simulink model "RO"  (R2023a)
settings: Solver=VariableStepAuto  StartTime=0.0  StopTime=10.0  RelTol=1e-3
undefined symbols (not defined in the file): SR
settings Model: Creator=mekala.suresh  LastModifiedBy=andres.lucht
settings OptimizationCC: ReuseModelBlockBuffer=off

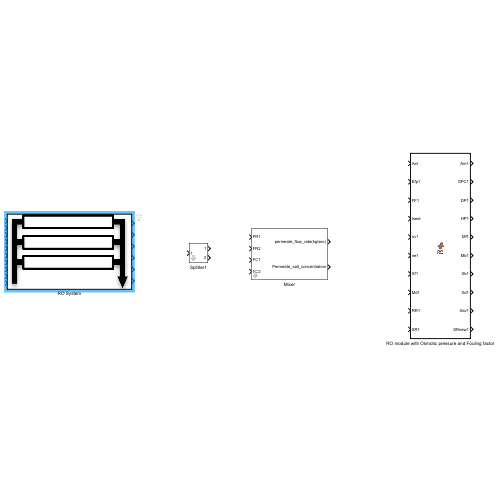
[thumbnail: Simulink's stored preview of the top-level diagram]
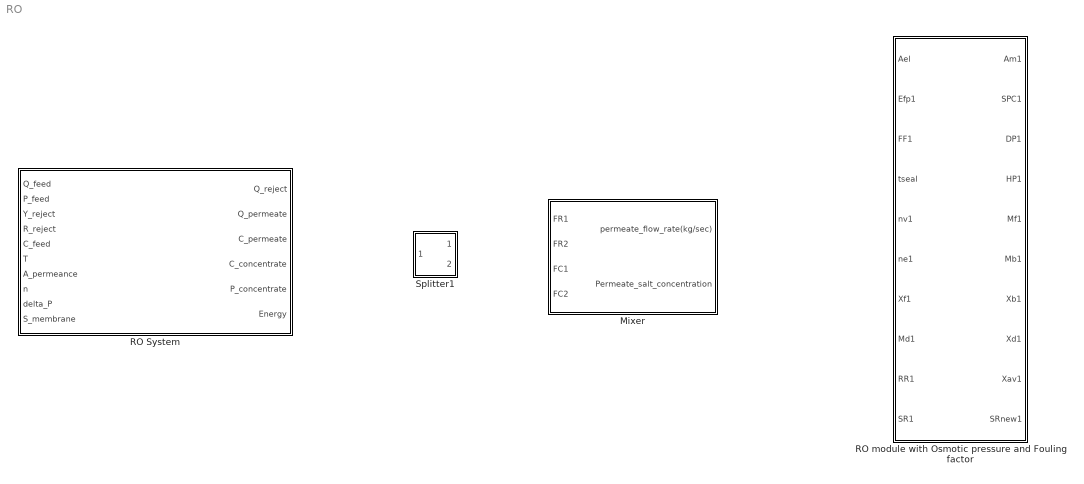
== system RO ==
  Mixer : Subsystem
      mask DialogControl DescTextVar Prompt: FR-Flow Rate
      mask DialogControl Control2 Prompt: FC-Flow Concentration
  RO System : MATLAB Function  TreatAsAtomicUnit=on
  RO module with Osmotic pressure and Fouling factor : MATLAB Function  TreatAsAtomicUnit=on
  Splitter1 : Subsystem  mask{Parameter2=0.750}
      mask prompts: Parameter2 "Split Ratio"
      mask DialogControl DescGroupVar Prompt: Splitter

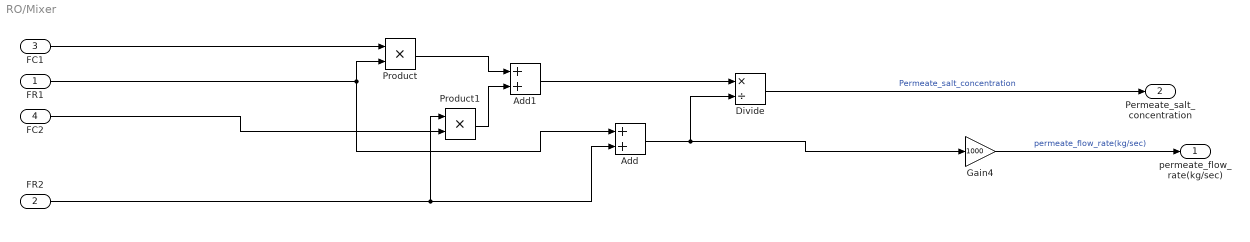
== system RO/Mixer ==
  FR1 : Inport
  FR2 : Inport  Port=2
  FC1 : Inport  Port=3
  FC2 : Inport  Port=4
  Add : Sum
  Add1 : Sum
  Divide : Product  Inputs=*/
  Gain4 : Gain  Gain=1000
  Product : Product
  Product1 : Product
  permeate_flow_rate(kg/sec) : Outport
  Permeate_salt_concentration : Outport  Port=2
  wires:
  Add/1 -> Gain4/1, Divide/2
  Divide/1 -> Permeate_salt_concentration/1  "Permeate_salt_concentration"
  Product/1 -> Add1/1
  Product1/1 -> Add1/2
  Add1/1 -> Divide/1
  Gain4/1 -> permeate_flow_rate(kg/sec)/1  "permeate_flow_rate(kg/sec)"
  FC2/1 -> Product1/2
  FC1/1 -> Product/1
  FR1/1 -> Add/1, Product/2
  FR2/1 -> Add/2, Product1/1

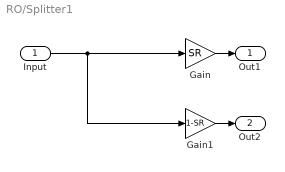
== system RO/Splitter1 ==
  Input : Inport
  Gain : Gain  Gain=SR
  Gain1 : Gain  Gain=1-SR
  Out1 : Outport
  Out2 : Outport  Port=2
  wires:
  Gain1/1 -> Out2/1
  Gain/1 -> Out1/1
  Input/1 -> Gain/1, Gain1/1

== matlab function RO/RO System ==
  data: Q_feed input; Q_reject output; P_feed input; Y_reject input; R_reject input; C_feed input; Q_permeate output; C_permeate output; C_concentrate output; P_concentrate output; T input; A_permeance input; n input; delta_P input; Energy output; S_membrane input
function [Q_reject,Q_permeate,C_permeate,C_concentrate,P_concentrate,Energy]  = RO_module(Q_feed,P_feed,Y_reject,R_reject,C_feed,T,A_permeance,n,delta_P,S_membrane)
% all the equations are derived from the mass balance of the desalination

% Copyright 2023 DECHEMA e.V., Theodor-Heuss-Allee 25, 60486 Frankfurt, Germany (https://dechema.de)
    % Contact: Andres Lucht Uribe
    % Developer: Suresh Mekala
    % Project H2Mare: https://www.wasserstoff-leitprojekte.de/projects/h2mare

% process
Q_reject = Q_feed .* Y_reject;                  % Concentrate flow rate
Q_permeate = Q_feed - Q_reject;                 % Permiate flow rate
C_permeate = (1 - R_reject) .* C_feed;          % permiate concentration
% Calculate salt concentration in the concentrate stream using mass balance
C_concentrate = ((Q_feed .* C_feed) - (Q_permeate .* C_permeate)) ./ Q_reject; % Concentrate concentration
I= 2;                                           %number of ions dissociated in the case of an electrolyte
% Concentration of salts in mol/m3
R = 8.314;                                      % ideal gas constant J/mol.K

delta_phi_osmotic = I * R * T .* (C_concentrate - C_permeate);  % osmotic pressure difference
A_water_permeance = A_permeance * exp(6.433 - 1885/T);          % m/s.Pa, water permeance constant
delta_P_p = ((delta_phi_osmotic) + (Q_permeate ./ (n*S_membrane*A_water_permeance))); % bar, transmembrane pressure drop
P_permeate = 1 ;                                                % P_feed - delta_P_transmembrane; % bar, permeate pressure
%P_reject = P_feed-(n*delta_P_transmembrane); % bar, concentrate pressure

P_concentrate = P_feed-delta_P ;

Energy = (((P_feed+P_concentrate)./2)*100)/(Y_reject.*0.8+3.6);

end

== matlab function RO/RO module with Osmotic pressure and Fouling factor ==
  data: Ael input; Am1 output; Efp1 input; FF1 input; tseal input; nv1 input; ne1 input; Xf1 input; Md1 input; RR1 input; SR1 input; SPC1 output; DP1 output; HP1 output; Mf1 output; Mb1 output; Xb1 output; Xd1 output; Xav1 output; SRnew1 output
function [Am1,SPC1,DP1,HP1,Mf1,Mb1,Xb1,Xd1,Xav1,SRnew1] = RO(Ael,Efp1,FF1,tseal,nv1,ne1,Xf1,Md1,RR1,SR1)

   %%%%%%% INPUTS %%%%%%%%%%%         |        %%%%%%%%% OUTPUTS%%%%%%%%%%%     |   
% Ael-    Element area m2             |      Am1 -  Total Membrabne Area        |        
% Efp1-   Pump efficiency             |      SPC1 - Specific Power consumption  | 
% FF1-    Fouling Factor              |      DP1 -  pressure diffeence          |
% t1 -    Ambinet temperature         |      HP1 -  Pump power                  | 
% tseal - Sea water temperature       |      Mf1 -  Feed water flow rate        | 
% nvl -   number of vessels           |      Mb1 -  brine flow rate             | 
% nel -   number of elements          |      Xb1 -  brine salinity              | 
% Xf1 -   Feed salinity kg/m3         |      Xd1 -  product salinity            | 
% Md1 -   Productivity feed           |      Xav1 - average salinity            | 
% RR1 -   permeate recovery rate      |      SEP1 - Specific entrophy production| 
% SR1 -   Salt Rejection rate         |      Irol1- Irreversibility             |
%                                     |      Ef1 -  Feed Exergy                 |
%                                     |      Eb1 -  Brine Exergy                | 
%                                     |      Ed1 -  Product Exergy              |
%                                     |      SRnew1-1st Salt rejection          |

%The permeate flow rate based on recovery ratio:
Mf1 = Md1./RR1;

% The paermeate salt concentration
Xd1 = Xf1.*(1-SR1);

%The rejected brine kg/s:
Mb1 = Mf1-Md1;

%the rejected salt concentration kg/m3;
Xb1 = ((Mf1.*Xf1)-(Md1.*Xd1))./Mb1;

%the average salt concentration kg/m3:
Xav1 = ((Mf1.*Xf1)+(Mb1.*Xb1))./(Mf1+Mb1);

%the temp correlation factor:
TCF = exp((8.859.*(tsel+273-298))./(tseal+273));

%the membrean water permeability:
kwr = (6.83.*(10^-8)).*((18.6865-(0.177.*Xb1))./(tseal+273));

kw = kwr;

%the salt permeability:

ksr = (4.72.*(10^-7)).*(0.06201-(5.31.*(10^-5).*(tseal+273)));
ks = ksr.*FF1.*TCF;

%calculation of osmotic pressure range(34.5~=75.84):

PAIf = 75.84.*Xf1;
PAIb = 75.84.*Xb1;
PAIp = 75.84.*Xd1;

%the average osmotic pressure acrross ion the feed side 
PAIav = 0.5.*(PAIf+PAIb);

%the net osmotic pressure across the membrane 
%SMW = 0.05833; %Where SMW is the salt molecular weight kg/kmol
%R = 8.314/1000 ; %universal gas constant kPA.m3/kMol.K
DPAI = PAIav - PAIp;

%the net pressure diference across the membrane:
DP1 = (Md1./(3600.*TCF.*FF1.*Ael.*ne1./nv1.*kw))+DPAI;

%the permeate area 
Am1 = Ae1.*ne1.*nv1;
Xdnew = (Am1.*3600.*ks.*(Xav1-Xd1))./Md1;

SRnew1 = 1-(Xdnew./Xf1);

%power required :
HP1=(100.*Mf1.*DP1)./(3600.*fraw(tseal,Xf1).*Efp1);

%specific power consumption:
SPC1 = HP1./Md1;




% 
% %Exergy Analysis:
% %%%%%%%%%%%%%%%%%%%%%%%%%%%%%%%%%%%%%%%%%%%%%%%%
% %If = ((1000.*Mb./3600).*(hf+hb))+((1000.*Mb./3600).*(hf-hb));
% Ms = 58.8;
% Mw=18;
% %%%%%%%%%%%%%%%%%%%%%%%%%%%%%%%%%%%%%%%%%%%%%%%%%%%%
% %Brine stream
% Npureb = (1000-Xb1)./Mw;
% Nsalt = Xb1./Ms;
% Nmb = Npureb+Nsaltb;
% 
% Xwb = Npureb./Nmb;
% Xsb = Nsalt./Nmb;
% 
% % Mmb = (Xsb*Ms)(Xwb*Mw);
% %echb = -Nmb.*(10^-3).*8.314.*(tsea+273).*((Xwb.*log(Xwb))+(Xsb.*log(Xsb));
% echb = Nmb.*(10^-3).*8.314.*(tsreal+273).*((-Xwb.*(log(Xwb)))-(Xsb.*(log(Xwb))));
% ephb = (fcp(t1,Xb1).*(t1-tseal))-(fcp(t1,Xb1).*tseal.*(log((t1+273)/(tseal+273))))+((DP1-275-101.1)./fraw(t1,Xb1));
% eb = ephb+echb;
% Eb1 = (Mb1.*1000./3600).*eb;
% 
% %%%%%%%%%%%%%%%%%%%%%%%%%%%%%%%%%
% %Feed stream:
% 
% Npuref = (1000-Xf1)./Mw;
% Nsaltf = Xf1./Ms;
% Nmf = Npuref+Nsaltf;
% 
% Xwf = Npuref./Nmf;
% Xsf = Nsaltf./Nmf;
% 
% %Mmf0=(Xsf*Ms)+(Xwf*Mw);
% 
% %echf =
% %-Nmf.*(10^-3).*8.314.*(tsea+273).*((Xwf.*log(Xwf))+(Xsf.*log(Xsf)));
% echf = Nmf.*(10^-3).*8.314.*(tseal+273).*((Xwf.*(log(Xwf)))-(Xsf.*(log(Xwf))));
% ephf = (fcp(t1,Xf1).*(t1-tseal))-fcp(t1,Xf1).*tseal.*(log((t1+273)/(tseal+273)))+((275-101.1)./fraw(t1,Xf1));
end
